simulink model "CK_index_bass"  (R2023a)
settings: Solver=VariableStepAuto  StartTime=0.0  StopTime=100  RelTol=1e-3
values from neighbouring files (symbols this model uses):
  a0 = 0.01    [script.m]
  a1 = 5    [script.m]
  a2 = 10    [script.m]
  a_i_notTop = 0    [script.m]
  a_i_Top = 1    [script.m]
  Alpha = 2    [script.m]
  Alpha1 = 10    [script.m]
  Alpha2 = 5    [script.m]
  Alpha3 = 1    [script.m]
  b0 = 0.001    [script.m]
  b1 = 0.25    [script.m]
  b2 = 1    [script.m]
  Cr = 1    [script.m]
  d1 = 0.1    [script.m]
  d2 = 1    [script.m]
  DCLV3 = 0.025    [script.m]
  DCLV3signal = 0.025    [script.m]
  DCyt = 0.25    [script.m]
  ds = 0.1    [script.m]
  DSstemcells = 0.025    [script.m]
  dw = 0.33    [script.m]
  K1 = 1    [script.m]
  K2 = 1    [script.m]
  Kh1 = 5    [script.m]
  Kh2 = 5    [script.m]
  n = 2    [script.m]
  ra = 0.025    [script.m]
  rclv = 0.025    [script.m]
  rclvs = 0.025    [script.m]
  rcyt = 0.025    [script.m]
  receptor_i1 = 0.01    [script.m]
  rsc = 0.025    [script.m]
  rw = 0.025    [script.m]
  V1 = 1    [script.m]
  Vh1 = 2    [script.m]
settings Model: Creator=mosuk  LastModifiedBy=mosuk

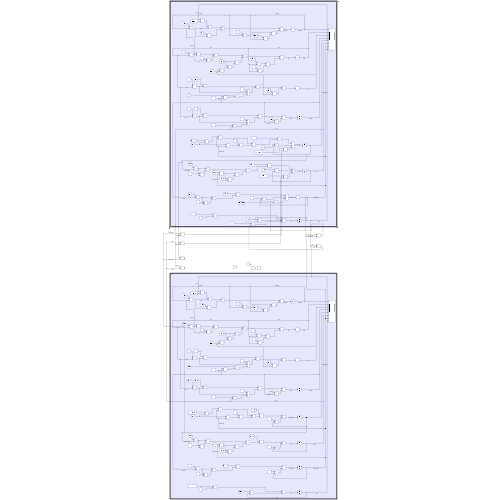
[thumbnail: Simulink's stored preview of the top-level diagram]
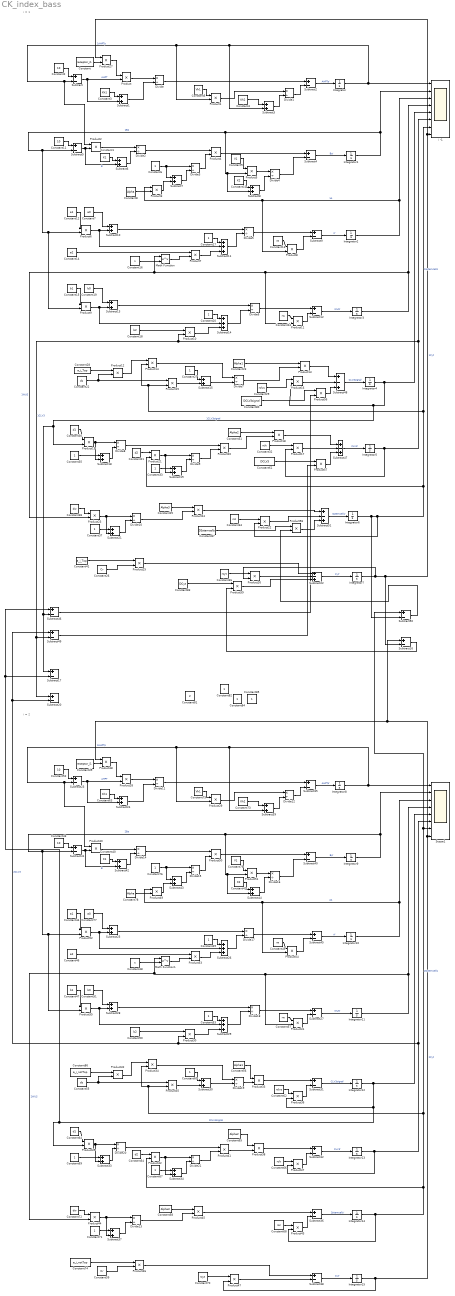
== system CK_index_bass ==
  note: i = 2
  note: i = 1
  Constant : Constant  Value=receptor_i1
  Constant1 : Constant  Value=K1
  Constant10 : Constant  Value=K2
  Constant{2,11,43,52} (4 alike) : Constant  Value=10
  Constant12 : Constant  Value=a1
  Constant13 : Constant  Value=ra
  Constant14 : Constant  Value=a2
  Constant15 : Constant  Value=b1
  Constant16 : Constant  Value=n
  Constant{6,17,20,27,33,35,37,49,53,60,67,69,71,76,82,84..85} (17 alike) : Constant
  Constant18 : Constant  Value=b2
  Constant19 : Constant  Value=b0
  Constant21 : Constant  Value=d2
  Constant22 : Constant  Value=ds
  Constant23 : Constant  Value=Alpha1
  Constant24 : Constant  Value=rw
  Constant25 : Constant  Value=Alpha3
  Constant26 : Constant  Value=Cr
  Constant28 : Constant  Value=a_i_Top
  Constant29 : Constant  Value=rclvs
  Constant3 : Constant  Value=Kh1
  Constant30 : Constant  Value=d1
  Constant31 : Constant  Value=Alpha2
  Constant32 : Constant  Value=rclv
  Constant34 : Constant  Value=rsc
  Constant36 : Constant  Value=rcyt
  Constant38 : Constant  Value=dw
  Constant39 : Constant  Value=receptor_i1
  Constant4 : Constant  Value=Kh2
  Constant40 : Constant  Value=K1
  Constant41 : Constant  Value=a_i_Top
  Constant42 : Constant  Value=K2
  Constant44 : Constant  Value=a1
  Constant45 : Constant  Value=ra
  Constant46 : Constant  Value=a2
  Constant47 : Constant  Value=b1
  Constant48 : Constant  Value=n
  Constant5 : Constant  Value=Vh1
  Constant50 : Constant  Value=b2
  Constant51 : Constant  Value=b0
  Constant54 : Constant  Value=d2
  Constant55 : Constant  Value=ds
  Constant56 : Constant  Value=Alpha1
  Constant57 : Constant  Value=rw
  Constant58 : Constant  Value=Alpha3
  Constant59 : Constant  Value=Cr
  Constant61 : Constant  Value=DCLV3
  Constant62 : Constant  Value=rclvs
  Constant63 : Constant  Value=Kh1
  Constant64 : Constant  Value=d1
  Constant65 : Constant  Value=Alpha2
  Constant66 : Constant  Value=rclv
  Constant68 : Constant  Value=rsc
  Constant7 : Constant  Value=a0
  Constant70 : Constant  Value=rcyt
  Constant72 : Constant  Value=dw
  Constant73 : Constant  Value=Kh2
  Constant74 : Constant  Value=a_i_notTop
  Constant75 : Constant  Value=Vh1
  Constant77 : Constant  Value=a0
  Constant78 : Constant  Value=Alpha
  Constant79 : Constant  Value=V1
  Constant8 : Constant  Value=Alpha
  Constant80 : Constant  Value=DCLV3signal
  Constant81 : Constant  Value=2
  Constant83 : Constant  Value=DCyt
  Constant86 : Constant  Value=a_i_notTop
  Constant87 : Constant  Value=DSstemcells
  Constant9 : Constant  Value=V1
  Divide{,1..21} (22 alike) : Product  Inputs=*/
  Integrator{,1..15} (16 alike) : Integrator
  Math Function : Math  Operator=pow
  Math Function1 : Math  Operator=pow
  Product{,1..59} (60 alike) : Product
  Scope1 : Scope  NumInputPorts=8
  Subtract{,2,4..5,9,12,16..17,20,23,27,31..32,35..36,38,40..41,45..46,49..50} (22 alike) : Sum  Inputs=+-
  Subtract{1,3,6..8,10,13,15,18..19,21,24..25,28,30,33..34,37,39,42..44} (22 alike) : Sum
  Subtract{11,14,26,29} (4 alike) : Sum  Inputs=+++
  Subtract{22,47..48,51} (4 alike) : Sum  Inputs=+-+
  i -1 : Scope  NumInputPorts=8
  wires:
  Product25/1 -> Subtract22/1
  Constant26/1 -> Product25/2
  Constant/1 -> Product27/2
  Constant17/1 -> Subtract11/1
  Product12/1 -> Product14/1
  Constant14/1 -> Product7/1
  Constant41/1 -> Product25/1
  Constant29/1 -> Product16/1
  Constant25/1 -> Product24/1
  Divide4/1 -> Subtract4/2
  Divide/1 -> Subtract2/1
  Divide9/1 -> Product20/2
  Product24/1 -> Subtract51/1
  Constant5/1 -> Product1/1
  Product19/1 -> Divide8/1, Subtract18/2
  Constant15/1 -> Product9/1
  Constant6/1 -> Subtract7/1, Divide3/1
  Subtract4/1 -> Integrator1/1  "Bp'"
  Subtract19/1 -> Divide9/2
  Constant13/1 -> Product8/1
  Constant34/1 -> Product22/1
  Subtract14/1 -> Divide6/2
  Subtract48/1 -> Integrator4/1  "CLV3signal'"
  Divide8/1 -> Product20/1
  Product17/1 -> Subtract47/2
  Divide10/1 -> Product24/2
  Subtract11/1 -> Divide5/2
  Product18/1 -> Subtract47/1
  Constant33/1 -> Subtract19/1
  Constant19/1 -> Subtract13/1
  Product23/1 -> Subtract21/2, Divide10/1
  Product1/1 -> Divide1/1
  Constant32/1 -> Product17/1
  Integrator2/1 -> Product8/2, Product3/1, i -1/3  "1A"
  Subtract2/1 -> Integrator/1  "AHPTp'"
  Constant36/1 -> Product26/1
  Divide1/1 -> Subtract2/2
  Product14/1 -> Divide7/1
  Subtract12/1 -> Integrator3/1  "WUS'"
  Product16/1 -> Subtract48/2
  Product26/1 -> Subtract22/2
  Subtract21/1 -> Divide10/2
  Subtract1/1 -> Divide/2
  Subtract8/1 -> Divide4/2
  Product3/1 -> Subtract7/2
  Product22/1 -> Subtract51/2
  Divide2/1 -> Product4/1
  Constant23/1 -> Product13/1
  Constant37/1 -> Subtract21/1
  Integrator6/1 -> Product21/2, Product15/2, Product14/2, i -1/7, Product22/2, Subtract50/2  "1Sstemcells"
  Constant28/1 -> Product12/1
  Math Function/1 -> Product7/2
  Constant22/1 -> Product12/2, Product15/1
  Product20/1 -> Product18/2
  Constant18/1 -> Product10/1
  Product21/1 -> Subtract19/2, Divide9/1
  Subtract5/1 -> Subtract6/2, Product2/2  "B"
  Constant2/1 -> Subtract/1
  Integrator7/1 -> Product26/2, Subtract16/2, Product27/1, i -1/8  "1Cyt"
  Constant8/1 -> Product3/2
  Constant21/1 -> Product21/1
  Product15/1 -> Subtract15/2
  Product4/1 -> Subtract4/1
  Product10/1 -> Subtract14/3
  Product5/1 -> Divide4/1
  Product9/1 -> Subtract14/2, Subtract13/2
  Constant31/1 -> Product18/1
  Divide7/1 -> Product13/2
  Integrator3/1 -> Product11/2, Product23/2, Math Function/1, i -1/4  "1WUS"
  Constant20/1 -> Subtract14/1
  Integrator4/1 -> i -1/5, Subtract17/1, Subtract46/2, Product19/2, Product16/2  "1CLV3signal"
  Integrator5/1 -> Product17/2, Subtract20/1, Subtract49/2, Product10/2, i -1/6  "1CLV3"
  Subtract15/1 -> Divide7/2
  Divide3/1 -> Product4/2
  Subtract6/1 -> Divide2/2
  Constant35/1 -> Subtract18/1
  Subtract13/1 -> Divide6/1
  Constant27/1 -> Subtract15/1
  Product8/1 -> Subtract9/2
  Constant3/1 -> Subtract1/1
  Product7/1 -> Subtract11/3
  Constant10/1 -> Subtract8/1
  Subtract/1 -> Subtract1/2, Product/2  "AHPT"
  Integrator1/1 -> i -1/2, Subtract8/2, Product5/2, Subtract5/2, Product9/2, Product6/2  "1Bp"
  Divide5/1 -> Subtract9/1
  Constant12/1 -> Product6/1
  Product27/1 -> Product/1
  Subtract10/1 -> Divide5/1
  Constant1/1 -> Subtract6/1
  Constant9/1 -> Product5/1
  Subtract9/1 -> Integrator2/1  "A'"
  Product13/1 -> Subtract48/1
  Integrator/1 -> Subtract3/2, Product1/2, Product2/1, Subtract/2, i -1/1  "1AHPTp"
  Subtract3/1 -> Divide1/2
  Product/1 -> Divide/1
  Subtract22/1 -> Integrator7/1  "Cyt'"
  Constant38/1 -> Product23/1
  Product11/1 -> Subtract12/2
  Divide6/1 -> Subtract12/1
  Subtract7/1 -> Divide3/2
  Constant24/1 -> Product11/1
  Constant4/1 -> Subtract3/1
  Constant7/1 -> Subtract10/1
  Product2/1 -> Divide2/1
  Constant16/1 -> Math Function/2
  Constant11/1 -> Subtract5/1
  Product6/1 -> Subtract11/2, Subtract10/2
  Subtract18/1 -> Divide8/2
  Constant30/1 -> Product19/1
  Product46/1 -> Subtract38/1
  Constant59/1 -> Product46/2
  Constant39/1 -> Product48/2
  Constant49/1 -> Subtract26/1
  Product32/1 -> Product34/1
  Constant46/1 -> Product53/1
  Constant74/1 -> Product46/1
  Constant62/1 -> Product36/1
  Constant58/1 -> Product45/1
  Divide16/1 -> Subtract40/2
  Divide11/1 -> Subtract35/1
  Divide21/1 -> Product41/2
  Product45/1 -> Subtract36/1
  Constant75/1 -> Product29/1
  Product39/1 -> Divide20/1, Subtract33/2
  Constant47/1 -> Product55/1
  Constant76/1 -> Subtract43/1, Divide15/1
  Subtract40/1 -> Integrator9/1  "Bp'"
  Subtract34/1 -> Divide21/2
  Constant45/1 -> Product54/1
  Constant68/1 -> Product43/1
  Subtract29/1 -> Divide18/2
  Subtract31/1 -> Integrator12/1  "CLV3signal'"
  Divide20/1 -> Product41/1
  Product37/1 -> Subtract32/2
  Divide13/1 -> Product45/2
  Subtract26/1 -> Divide17/2
  Product38/1 -> Subtract32/1
  Constant67/1 -> Subtract34/1
  Constant51/1 -> Subtract28/1
  Product44/1 -> Subtract37/2, Divide13/1
  Subtract32/1 -> Integrator13/1  "CLV3'"
  Product29/1 -> Divide12/1
  Constant66/1 -> Product37/1
  Integrator10/1 -> Product54/2, Product49/1, Scope1/3  "2A"
  Subtract35/1 -> Integrator8/1  "AHPTp'"
  Constant70/1 -> Product47/1
  Divide12/1 -> Subtract35/2
  Product34/1 -> Divide19/1
  Subtract27/1 -> Integrator11/1  "WUS'"
  Product36/1 -> Subtract31/2
  Product47/1 -> Subtract38/2
  Subtract37/1 -> Divide13/2
  Subtract24/1 -> Divide11/2
  Subtract44/1 -> Divide16/2
  Product49/1 -> Subtract43/2
  Product43/1 -> Subtract36/2
  Divide14/1 -> Product50/1
  Constant56/1 -> Product33/1
  Constant71/1 -> Subtract37/1
  Integrator14/1 -> Product43/2, Product42/2, Product35/2, Product34/2, Subtract50/1, Scope1/7  "2Sstemcells"
  Constant86/1 -> Product32/1
  Math Function1/1 -> Product53/2
  Constant55/1 -> Product32/2, Product35/1
  Product41/1 -> Product38/2
  Constant50/1 -> Product30/1
  Product42/1 -> Subtract34/2, Divide21/1
  Subtract41/1 -> Subtract42/2, Product40/2  "B"
  Constant52/1 -> Subtract23/1
  Integrator15/1 -> Product47/2, Subtract16/1, Product48/1, Scope1/8  "2Cyt"
  Constant78/1 -> Product49/2
  Constant54/1 -> Product42/1
  Product35/1 -> Subtract30/2
  Product50/1 -> Subtract40/1
  Product30/1 -> Subtract29/3
  Product51/1 -> Divide16/1
  Product55/1 -> Subtract29/2, Subtract28/2
  Constant65/1 -> Product38/1
  Divide19/1 -> Product33/2
  Integrator11/1 -> Product31/2, Product44/2, Math Function1/1, Scope1/4  "2WUS"
  Constant53/1 -> Subtract29/1
  Integrator12/1 -> Subtract17/2, Subtract46/1, Product39/2, Product36/2, Scope1/5  "2CLV3signal"
  Integrator13/1 -> Subtract20/2, Subtract49/1, Product30/2, Scope1/6, Product37/2  "2CLV3"
  Subtract30/1 -> Divide19/2
  Divide15/1 -> Product50/2
  Subtract42/1 -> Divide14/2
  Constant69/1 -> Subtract33/1
  Subtract28/1 -> Divide18/1
  Constant60/1 -> Subtract30/1
  Product54/1 -> Subtract45/2
  Constant63/1 -> Subtract24/1
  Product53/1 -> Subtract26/3
  Constant42/1 -> Subtract44/1
  Subtract23/1 -> Subtract24/2, Product28/2  "AHPT"
  Integrator9/1 -> Scope1/2, Subtract44/2, Product51/2, Subtract41/2, Product55/2, Product52/2  "2Bp"
  Divide17/1 -> Subtract45/1
  Constant44/1 -> Product52/1
  Product48/1 -> Product28/1
  Subtract25/1 -> Divide17/1
  Constant40/1 -> Subtract42/1
  Constant79/1 -> Product51/1
  Subtract45/1 -> Integrator10/1  "A'"
  Product33/1 -> Subtract31/1
  Integrator8/1 -> Subtract39/2, Product29/2, Product40/1, Subtract23/2, Scope1/1  "2AHPTp"
  Subtract39/1 -> Divide12/2
  Product28/1 -> Divide11/1
  Subtract38/1 -> Integrator15/1  "Cyt'"
  Constant72/1 -> Product44/1
  Product31/1 -> Subtract27/2
  Divide18/1 -> Subtract27/1
  Subtract43/1 -> Divide15/2
  Constant57/1 -> Product31/1
  Constant73/1 -> Subtract39/1
  Subtract36/1 -> Integrator14/1  "Sstemcells'"
  Constant77/1 -> Subtract25/1
  Product40/1 -> Divide14/1
  Constant48/1 -> Math Function1/2
  Constant43/1 -> Subtract41/1
  Product52/1 -> Subtract26/2, Subtract25/2
  Subtract33/1 -> Divide20/2
  Constant64/1 -> Product39/1
  Subtract46/1 -> Product56/2
  Constant80/1 -> Product56/1
  Subtract47/1 -> Integrator5/1  "CLV3'"
  Product56/1 -> Subtract48/3
  Product57/1 -> Subtract47/3
  Constant61/1 -> Product57/1
  Subtract49/1 -> Product57/2
  Subtract51/1 -> Integrator6/1  "Sstemcells'"
  Constant87/1 -> Product58/1
  Subtract50/1 -> Product58/2
  Product58/1 -> Subtract51/3
  Constant83/1 -> Product59/1
  Product59/1 -> Subtract22/3
  Subtract16/1 -> Product59/2
